simulink model "eight_model"  (R2022a)
settings: Solver=FixedStepAuto  StartTime=0.0  StopTime=10.0  FixedStep=1e-3  RelTol=1e-3  EnableMultiTasking=on
undefined symbols (not defined in the file): D0, D1, D10, D11, D12, D13, D2, D3, D4, D5, D6, D7, D8, D9, magnitude, PTA0, PTA1, PTA2, PTB23, PTB9, PTC16, PTC17, PTC2, PTC3, PTC4, PTD0, PTD1, PTD2, PTD3
libraries: etargetslib x30, frdmk64flib x18, dspstat3 x1, simulink x1
settings Model: ExtModeTrigDuration=5  Creator=12791  LastModifiedBy=12791
settings OptimizationCC: EnhancedBackFolding=on  PassReuseOutputArgsAs=Individual arguments  ZeroExternalMemoryAtStartup=off  ZeroInternalMemoryAtStartup=off  MaxStackSize=64  OptimizeBlockOrder=speed  DifferentSizesBufferReuse=on  OptimizationCustomize=off  EfficientTunableParamExpr=on
settings DebuggingCC: ParameterTunabilityLossMsg=error
settings HardwareCC: ProdBitPerPointer=32  ProdBitPerSizeT=32  ProdBitPerPtrDiffT=32  ProdLargestAtomicInteger=Long  ProdLargestAtomicFloat=Double  ProdWordSize=32  ProdHWDeviceType=ARM Compatible->ARM Cortex
settings SFSimCC: MATLABDynamicMemAlloc=off
settings RTWCC: SystemTargetFile=ert.tlc  HardwareBoard=NXP FRDM-K64F  TLCOptions="-aInlineSetEventsForThisBaseRateFcn=TLC_FALSE -aSuppressMultiTaskScheduler=TLC_FALSE  -aRateBasedStepFcn=0"  TemplateMakefile=ert_default_tmf  Toolchain=GNU Tools for ARM Embedded Processors
settings CodeAppCC: ForceParamTrailComments=on  IgnoreCustomStorageClasses=off  OperatorAnnotations=on  SimulinkDataObjDesc=on  SFDataObjDesc=on  InsertBlockDesc=on
settings ERTTargetCC: ExtModeTransport=4  ExtModeMexFile=sendToCommService

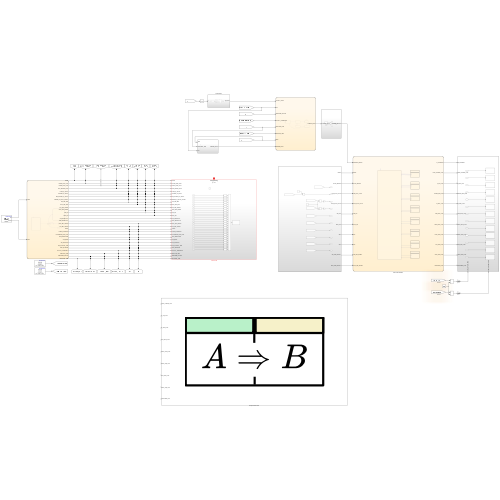
[thumbnail: Simulink's stored preview of the top-level diagram]
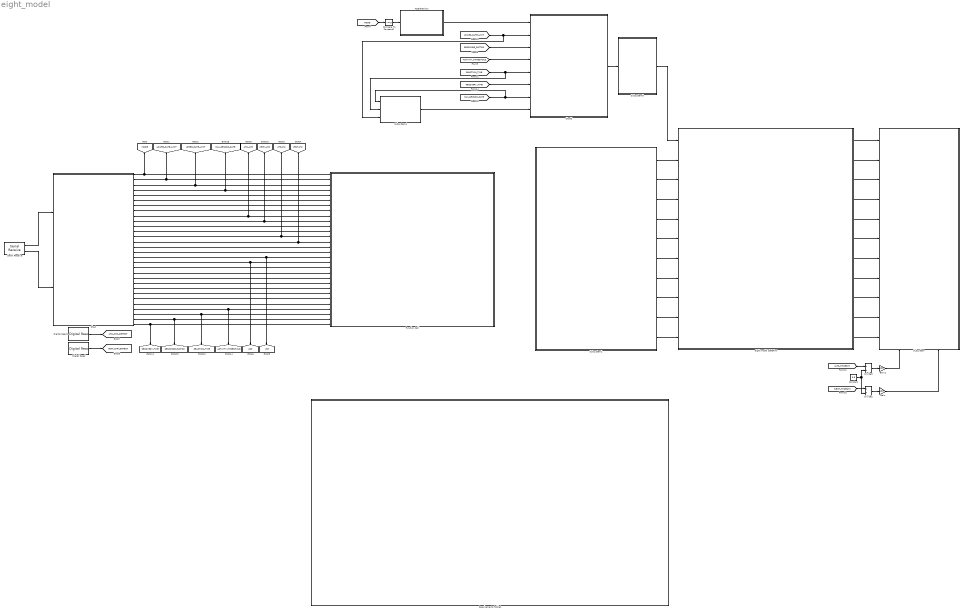
== system eight_model ==
  Acceleration1 : Subsystem
  Chart : Stateflow chart  TreatAsAtomicUnit=on
  Chart2 : Stateflow chart  TreatAsAtomicUnit=on
  Compare To Constant2 : simulink/Logic and Bit Operations/Compare To Constant  relop=>=  const=5  OutDataTypeStr=boolean
  Constant : Constant  Value=3.3
  Digital Read : frdmk64flib/Digital Read  Whichpin=PTC17 (D1)  SampleTime=-1
  Digital Read1 : frdmk64flib/Digital Read  Whichpin=PTC16 (D0)  SampleTime=-1
  Divide2 : Product  Inputs=*/
  Divide3 : Product  Inputs=*/
  Function Call : Subsystem  TreatAsAtomicUnit=on
  Gain : Gain  Gain=100
  Gain1 : Gain  Gain=100
  Requirements Table1 : Requirements Table  TreatAsAtomicUnit=on
  Serial Receive : frdmk64flib/Serial Receive  SCIModule=0  Baudrate=uint32(9600)  Parity=None  StopBits=1  HardwareFlowControl=None  ByteOrder=LittleEndian  DataType=uint8  DataLength=10  BlockingMode=off  OutputStatus=on  SampleTime=0.1
  Subsystem : Subsystem
      settings: PortSchema="{\"entries\":[{\"content\":{\"sides\":[{\"content\":{\"connectorIds\":[\"In1\",\"In2\",\"In3\",\"In4\",\"In5\",\"In6\",\"In7\",\"In8\",\"In9\",\"In10\",\"In11\"]},\"type\":\"ConnectorPlacement.EquallySpacedRectSide\",\"uuid\":\"cf431d19-a261-4061-b975-82ab8e4554ba\"},{\"content\":{\"connectorIds\":[],\"side\":\"RIGHT\"},\"type\":\"ConnectorPlacement.EquallySpacedRectSide\",\"uuid\":\"d9d96e0a-6018-4f8e-a98f-6eed3a91414e\"},{\"content\":{\"connectorIds\":[],\"side\":\"TOP\"},\"type\":\"ConnectorPlacement.EquallySpacedRectSide\",\"uuid\":\"2358aaff-c3a0-4959-bedb-835f64f1bbed\"},{\"content\":{\"connectorIds\":[\"In12\",\"In13\"],\"side\":\"BOTTOM\"},\"type\":\"ConnectorPlacement.EquallySpacedRectSide\",\"uuid\":\"ece4eb5b-308d-4002-b014-99ad51b61e06\"}]},\"type\":\"ConnectorPlacement.EquallySpacedConnector\",\"uuid\":\"cdbd5127-fb13-4f48-9ecc-e21d40fbaa52\"}],\"packageUris\":[\"http://schema.mathworks.com/mf0/Connector/R2020b\"],\"version\":\"1.0\"}"
  Subsystem1 : Subsystem
  Subsystem4 : Subsystem
  Subsystem5 : Subsystem
  eight model stateflow : Stateflow chart  TreatAsAtomicUnit=on
      settings: PortSchema="{\"entries\":[{\"content\":{\"sides\":[{\"content\":{\"connectorIds\":[\"In6\",\"In7\",\"In2\",\"In4\",\"In1\",\"In8\",\"In9\",\"In11\",\"In10\",\"In5\",\"In3\"]},\"type\":\"ConnectorPlacement.EquallySpacedRectSide\",\"uuid\":\"7bd189cb-d286-447b-b347-38d7b12e59ee\"},{\"content\":{\"connectorIds\":[\"Out1\",\"Out2\",\"Out3\",\"Out4\",\"Out5\",\"Out6\",\"Out7\",\"Out8\",\"Out9\",\"Out10\",\"Out11\"],\"side\":\"RIGHT\"},\"type\":\"ConnectorPlacement.EquallySpacedRectSide\",\"uuid\":\"522f4543-8a7d-441b-9c0c-141bccf5cf26\"},{\"content\":{\"connectorIds\":[],\"side\":\"TOP\"},\"type\":\"ConnectorPlacement.EquallySpacedRectSide\",\"uuid\":\"cf7ae06b-6ef3-498b-825a-38a0a4c90c8a\"}]},\"type\":\"ConnectorPlacement.EquallySpacedConnector\",\"uuid\":\"ae15f7ff-4998-48cc-acd9-270deb6c013f\"}],\"packageUris\":[\"http://schema.mathworks.com/mf0/Connector/R2020b\"],\"version\":\"1.0\"}"
  tag scope: ACTIVITY_THRESHOLD=global, ARP=global, ATR_AMP=global, ATR_CMP_DETECT=global, ATR_PW=global, LOWER_RATE_LIMIT=global, MAX_SENSOR_RATE=global, MODE=global, REACTION_TIME=global, RECOVERY_TIME=global, RESPONSE_FACTOR=global, UPPER_RATE_LIMIT=global, VENT_AMP=global, VENT_CMP_DETECT=global, VENT_PW=global, VRP=global
  wires:
  eight model stateflow/1(IS_CHARGING) -> Subsystem/1(IS_CHARGING)
  eight model stateflow/2(PACE_CHARGE_CTRL) -> Subsystem/2(PACE_CHARGE_CTRL)
  eight model stateflow/3(Z_ATR_CTRL) -> Subsystem/3(Z_ATR_CTRL)
  eight model stateflow/4(PACING_REF_PWM) -> Subsystem/4(PACING_REF_PWM)
  eight model stateflow/5(Z_VENT_CTRL) -> Subsystem/5(Z_VENT_CTRL)
  eight model stateflow/6(ATR_PACE_CTRL) -> Subsystem/6(ATR_PACE_CTRL)
  eight model stateflow/7(VENT_PACE_CTRL) -> Subsystem/7(VENT_PACE_CTRL)
  eight model stateflow/8(PACE_GND_CTRL) -> Subsystem/8(PACE_GND_CTRL)
  eight model stateflow/9(ATR_GND_CTRL) -> Subsystem/9(ATR_GND_CTRL)
  eight model stateflow/10(VENT_GND_CTRL) -> Subsystem/10(VENT_GND_CTRL)
  eight model stateflow/11(FRONTEND_CTRL) -> Subsystem/11(FRONTEND_CTRL)
  Serial Receive/1 -> Chart/1(rxdata)
  Serial Receive/2 -> Chart/2(status)
  Chart/1(MODE) -> Function Call/1(MODE), [MODE]
  Chart/2(LOWER_RATE_LIMIT) -> Function Call/2(LOWER_RATE_LIMIT), [LOWER_RATE_LIMIT]
  Chart/3(UPPER_RATE_LIMIT) -> Function Call/3(UPPER_RATE_LIMIT), [UPPER_RATE_LIMIT]
  Chart/4(MAX_SENSOR_RATE) -> Function Call/4(MAX_SENSOR_RATE), [MAX_SENSOR_RATE]
  Chart/5(FIXED_AV_DELAY) -> Function Call/5(FIXED_AV_DELAY)
  Chart/6(DYNAMIC_AV_DELAY) -> Function Call/6(DYNAMIC_AV_DELAY)
  Chart/7(MIN_DYNAMIC_AV_DELAY) -> Function Call/7(MIN_DYNAMIC_AV_DELAY)
  Chart/8(SENSED_AV_DELAY_OFFSET) -> Function Call/8(SENSED_AV_DELAY_OFFSET)
  Chart/11(ATR_AMP_UNREG) -> Function Call/11(ATR_AMP_UNREG)
  Chart/12(VENT_AMP_UNREG) -> Function Call/12(VENT_AMP_UNREG)
  Chart/13(ATR_PW) -> Function Call/13(ATR_PW), [ATR_PW]
  Chart/14(VENT_PW) -> Function Call/14(VENT_PW), [VENT_PW]
  Chart/15(ATR_SENSITIVITY) -> Function Call/15(ATR_SENSITIVITY)
  Chart/16(VENT_SENSITIVITY) -> Function Call/16(VENT_SENSITIVITY)
  Chart/17(VENT_REF_PERIOD) -> Function Call/17(VENT_REF_PERIOD), [VRP]
  Chart/18(ATR_REF_PERIOD) -> Function Call/18(ATR_REF_PERIOD), [ARP]
  Chart/19(PVARP) -> Function Call/19(PVARP)
  Chart/20(PVARP_EXTENSION) -> Function Call/20(PVARP_EXTENSION)
  Chart/21(HYSTERESIS_RATE_LIMIT) -> Function Call/21(HYSTERESIS_RATE_LIMIT)
  Chart/22(RATE_SMOOTHING) -> Function Call/22(RATE_SMOOTHING)
  Chart/23(ATR_MODE) -> Function Call/23(ATR_MODE)
  Chart/24(ATR_DURATION) -> Function Call/24(ATR_DURATION)
  Chart/25(ATR_FALLBACK_TIME) -> Function Call/25(ATR_FALLBACK_TIME)
  Chart/26(VENT_BLANKING) -> Function Call/26(VENT_BLANKING)
  Chart/27(ACTIVITY_THRESHOLD) -> [ACTIVITY_THRESHOLD], Function Call/27(ACTIVITY_THRESHOLD)
  Chart/29(RESPONSE_FACTOR) -> Function Call/29(RESPONSE_FACTOR), [RESPONSE_FACTOR]
  Chart/30(RECOVERY_TIME) -> Function Call/30(RECOVERY_TIME), [RECOVERY_TIME]
  Subsystem1/2(PULSE_PERIOD) -> eight model stateflow/2(PULSE_PERIOD)
  Subsystem1/1(MODE) -> eight model stateflow/7(MODE)
  Subsystem1/4(VENT_DUTY_CYCLE) -> eight model stateflow/1(VENT_DUTY_CYCLE)
  Subsystem1/5(ATR_PW) -> eight model stateflow/8(ATR_PW)
  Subsystem1/6(VENT_PW) -> eight model stateflow/9(VENT_PW)
  Subsystem1/7(ARP) -> eight model stateflow/11(ARP)
  Subsystem1/8(VRP) -> eight model stateflow/10(VRP)
  Subsystem1/3(ATR_DUTY_CYCLE) -> eight model stateflow/4(ATR_DUTY_CYCLE)
  Subsystem1/9(ATR_CMP_DETECT) -> eight model stateflow/5(ATR_CMP_DETECT)
  Subsystem1/10(VENT_CMP_DETECT) -> eight model stateflow/3(VENT_CMP_DETECT)
  Divide2/1 -> Gain/1
  Divide3/1 -> Gain1/1
  Constant/1 -> Divide2/2, Divide3/2
  [VENT_THRESH] -> Divide2/1
  [ATR_THRESH] -> Divide3/1
  Gain/1 -> Subsystem/13(VENT_CMP_REF_PWM)
  Gain1/1 -> Subsystem/12(ATR_CMP_REF_PWM)
  Digital Read1/1 -> [ATR_CMP_DETECT]
  Digital Read/1 -> [VENT_CMP_DETECT]
  Chart/10(VENT_AMP_REG) -> Function Call/10(VENT_AMP_REG), [VENT_AMP]
  Chart/9(ATR_AMP_REG) -> Function Call/9(ATR_AMP_REG), [ATR_AMP]
  Chart/28(REACTION_TIME) -> Function Call/28(REACTION_TIME), [REACTION_TIME]
  [RESPONSE_FACTOR] -> Chart2/3(RESPONSE_FACTOR)
  Chart2/1(CURRENT_RATE) -> Subsystem5/1(CURRENT_RATE)
  [LOWER_RATE_LIMIT] -> Subsystem4/3(LRL), Chart2/2(LRL)
  Subsystem4/1(DESIRED_RATE) -> Chart2/8(DESIRED_RATE)
  [REACTION_TIME] -> Subsystem4/2(RESPONSE_TIME), Chart2/5(REACTION_TIME)
  [MAX_SENSOR_RATE] -> Subsystem4/1(MSR), Chart2/7(MSR)
  [MODE] -> Compare To Constant2/1
  Compare To Constant2/1 -> Acceleration1/1(In1)
  [ACTIVITY_THRESHOLD] -> Chart2/4(ACTIVITY_THRESHOLD)
  Acceleration1/1(ACTIVITY) -> Chart2/1(ACTIVITY_LEVEL)
  [RECOVERY_TIME] -> Chart2/6(RECOVER_TIME)
  Subsystem5/1(MODIFIED_PERIOD) -> eight model stateflow/6(MODIFIED_PERIOD)

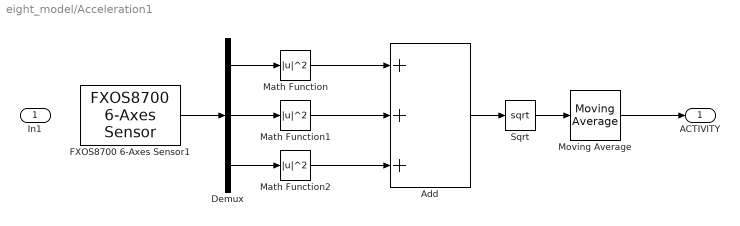
== system eight_model/Acceleration1 ==
  In1 : Inport
  Add : Sum  Inputs=+++
  Demux : Demux  Outputs=3
  FXOS8700 6-Axes Sensor1 : frdmk64flib/FXOS8700 6-Axes Sensor  Activesensor=Accelerometer only  ODR=800Hz  HybridODR=400Hz  Accelfullrange=-4g to +4g  SampleTime=-1
  Math Function : Math  Operator=magnitude^2  SignedPower=on  OutDataTypeStr=double
  Math Function1 : Math  Operator=magnitude^2  SignedPower=on  OutDataTypeStr=double
  Math Function2 : Math  Operator=magnitude^2  SignedPower=on  OutDataTypeStr=double
  Moving Average : dspstat3/Moving Average  Method=Sliding window  ForgettingFactorPort=off  SpecifyWindowLength=on  WindowLength=4  ForgettingFactor=0.9  SimulateUsing=Code generation
  Sqrt : Sqrt
  ACTIVITY : Outport  SourceOfInitialOutputValue=Input signal
  wires:
  Sqrt/1 -> Moving Average/1
  Math Function2/1 -> Add/3
  Add/1 -> Sqrt/1
  Math Function1/1 -> Add/2
  Demux/1 -> Math Function/1
  Demux/2 -> Math Function1/1
  Math Function/1 -> Add/1
  FXOS8700 6-Axes Sensor1/1 -> Demux/1
  Demux/3 -> Math Function2/1
  Moving Average/1 -> ACTIVITY/1

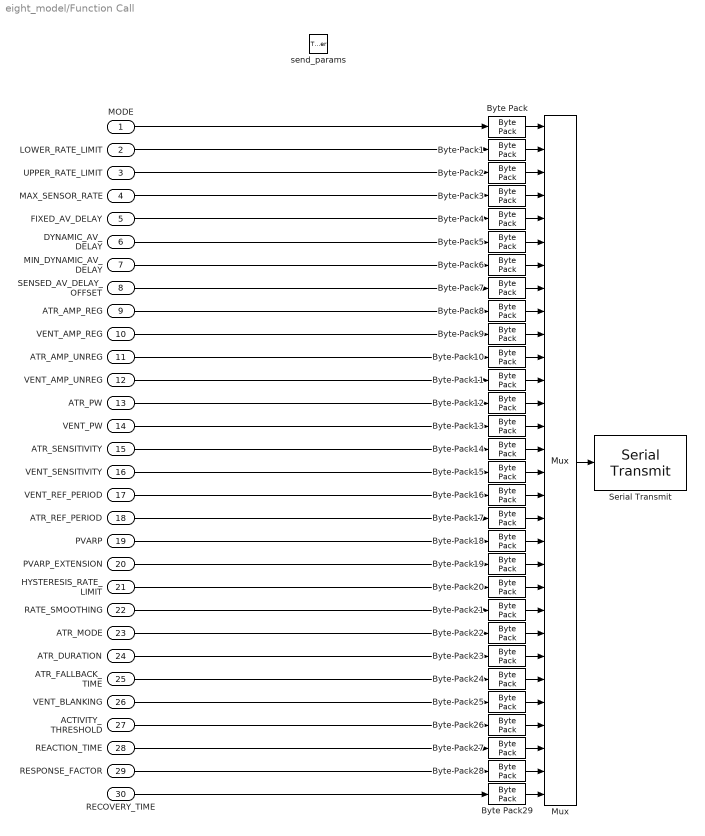
== system eight_model/Function Call ==
  MODE : Inport
  LOWER_RATE_LIMIT : Inport  Port=2
  UPPER_RATE_LIMIT : Inport  Port=3
  MAX_SENSOR_RATE : Inport  Port=4
  FIXED_AV_DELAY : Inport  Port=5
  DYNAMIC_AV_DELAY : Inport  Port=6
  MIN_DYNAMIC_AV_DELAY : Inport  Port=7
  SENSED_AV_DELAY_OFFSET : Inport  Port=8
  ATR_AMP_REG : Inport  Port=9
  VENT_AMP_REG : Inport  Port=10
  ATR_AMP_UNREG : Inport  Port=11
  VENT_AMP_UNREG : Inport  Port=12
  ATR_PW : Inport  Port=13
  VENT_PW : Inport  Port=14
  ATR_SENSITIVITY : Inport  Port=15
  VENT_SENSITIVITY : Inport  Port=16
  VENT_REF_PERIOD : Inport  Port=17
  ATR_REF_PERIOD : Inport  Port=18
  PVARP : Inport  Port=19
  PVARP_EXTENSION : Inport  Port=20
  HYSTERESIS_RATE_LIMIT : Inport  Port=21
  RATE_SMOOTHING : Inport  Port=22
  ATR_MODE : Inport  Port=23
  ATR_DURATION : Inport  Port=24
  ATR_FALLBACK_TIME : Inport  Port=25
  VENT_BLANKING : Inport  Port=26
  ACTIVITY_THRESHOLD : Inport  Port=27
  REACTION_TIME : Inport  Port=28
  RESPONSE_FACTOR : Inport  Port=29
  RECOVERY_TIME : Inport  Port=30
  send_params : TriggerPort  TriggerType=function-call  IsSimulinkFunction=on  FunctionName=send_params  VariantControl=Variant
  Byte Pack{,1..4,6..7,16..21,23..25,27..29} (19 alike) : etargetslib/Byte Pack  datatypes={'uint16'}  byteAlign=1
  Byte Pack{8..15,26} (9 alike) : etargetslib/Byte Pack  datatypes={'double'}  byteAlign=1
  Byte Pack22 : etargetslib/Byte Pack  datatypes={'boolean'}  byteAlign=1
  Byte Pack5 : etargetslib/Byte Pack  datatypes={'boolean'}  byteAlign=1
  Mux : Mux  Inputs=30
  Serial Transmit : frdmk64flib/Serial Transmit  SCIModule=0  Baudrate=uint32(9600)  Parity=None  StopBits=1  HardwareFlowControl=None  ByteOrder=LittleEndian  BlockingMode=on  OutputStatus=off
  wires:
  PVARP/1 -> Byte Pack18/1
  ATR_SENSITIVITY/1 -> Byte Pack14/1
  PVARP_EXTENSION/1 -> Byte Pack19/1
  MAX_SENSOR_RATE/1 -> Byte Pack3/1
  Byte Pack1/1 -> Mux/2
  Byte Pack7/1 -> Mux/8
  Byte Pack21/1 -> Mux/22
  ATR_AMP_UNREG/1 -> Byte Pack10/1
  Byte Pack/1 -> Mux/1
  Byte Pack20/1 -> Mux/21
  Byte Pack22/1 -> Mux/23
  Byte Pack3/1 -> Mux/4
  Byte Pack18/1 -> Mux/19
  VENT_REF_PERIOD/1 -> Byte Pack16/1
  Byte Pack17/1 -> Mux/18
  Mux/1 -> Serial Transmit/1
  Byte Pack26/1 -> Mux/27
  Byte Pack12/1 -> Mux/13
  LOWER_RATE_LIMIT/1 -> Byte Pack1/1
  RECOVERY_TIME/1 -> Byte Pack29/1
  Byte Pack9/1 -> Mux/10
  Byte Pack19/1 -> Mux/20
  Byte Pack13/1 -> Mux/14
  RESPONSE_FACTOR/1 -> Byte Pack28/1
  ATR_DURATION/1 -> Byte Pack23/1
  RATE_SMOOTHING/1 -> Byte Pack21/1
  Byte Pack8/1 -> Mux/9
  REACTION_TIME/1 -> Byte Pack27/1
  Byte Pack29/1 -> Mux/30
  Byte Pack16/1 -> Mux/17
  Byte Pack25/1 -> Mux/26
  ATR_MODE/1 -> Byte Pack22/1
  VENT_SENSITIVITY/1 -> Byte Pack15/1
  Byte Pack11/1 -> Mux/12
  VENT_PW/1 -> Byte Pack13/1
  MODE/1 -> Byte Pack/1
  VENT_AMP_REG/1 -> Byte Pack9/1
  Byte Pack24/1 -> Mux/25
  Byte Pack15/1 -> Mux/16
  Byte Pack2/1 -> Mux/3
  MIN_DYNAMIC_AV_DELAY/1 -> Byte Pack6/1
  VENT_BLANKING/1 -> Byte Pack25/1
  Byte Pack28/1 -> Mux/29
  ATR_PW/1 -> Byte Pack12/1
  FIXED_AV_DELAY/1 -> Byte Pack4/1
  VENT_AMP_UNREG/1 -> Byte Pack11/1
  Byte Pack4/1 -> Mux/5
  UPPER_RATE_LIMIT/1 -> Byte Pack2/1
  Byte Pack27/1 -> Mux/28
  SENSED_AV_DELAY_OFFSET/1 -> Byte Pack7/1
  Byte Pack6/1 -> Mux/7
  ATR_AMP_REG/1 -> Byte Pack8/1
  Byte Pack14/1 -> Mux/15
  Byte Pack10/1 -> Mux/11
  DYNAMIC_AV_DELAY/1 -> Byte Pack5/1
  Byte Pack5/1 -> Mux/6
  ATR_REF_PERIOD/1 -> Byte Pack17/1
  ACTIVITY_THRESHOLD/1 -> Byte Pack26/1
  Byte Pack23/1 -> Mux/24
  HYSTERESIS_RATE_LIMIT/1 -> Byte Pack20/1
  ATR_FALLBACK_TIME/1 -> Byte Pack24/1

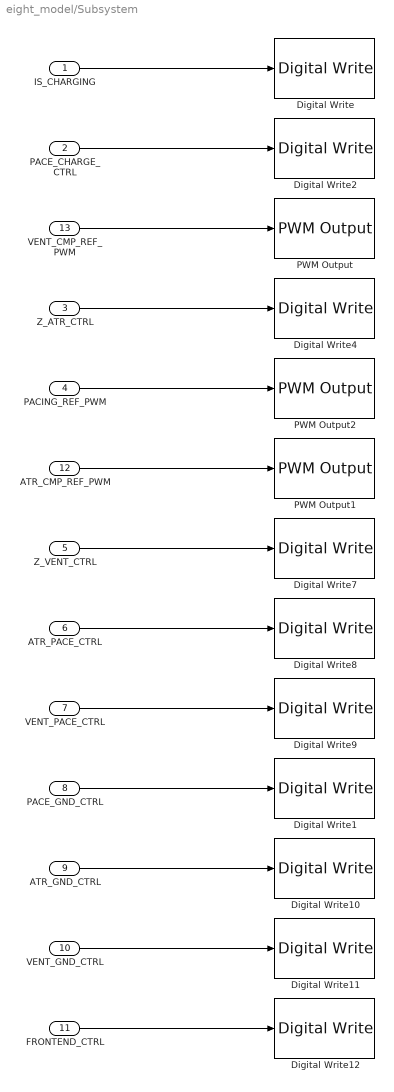
== system eight_model/Subsystem ==
  IS_CHARGING : Inport
  PACE_CHARGE_CTRL : Inport  Port=2
  Z_ATR_CTRL : Inport  Port=3
  PACING_REF_PWM : Inport  Port=4
  Z_VENT_CTRL : Inport  Port=5
  ATR_PACE_CTRL : Inport  Port=6
  VENT_PACE_CTRL : Inport  Port=7
  PACE_GND_CTRL : Inport  Port=8
  ATR_GND_CTRL : Inport  Port=9
  VENT_GND_CTRL : Inport  Port=10
  FRONTEND_CTRL : Inport  Port=11
  ATR_CMP_REF_PWM : Inport  Port=12
  VENT_CMP_REF_PWM : Inport  Port=13
  Digital Write : frdmk64flib/Digital Write  Whichpin=RED_LED
  Digital Write1 : frdmk64flib/Digital Write  Whichpin=PTD0 (D10)
  Digital Write10 : frdmk64flib/Digital Write  Whichpin=PTD2 (D11)
  Digital Write11 : frdmk64flib/Digital Write  Whichpin=PTD3 (D12)
  Digital Write12 : frdmk64flib/Digital Write  Whichpin=PTD1 (D13)
  Digital Write2 : frdmk64flib/Digital Write  Whichpin=PTB9 (D2)
  Digital Write4 : frdmk64flib/Digital Write  Whichpin=PTB23 (D4)
  Digital Write7 : frdmk64flib/Digital Write  Whichpin=PTC3 (D7)
  Digital Write8 : frdmk64flib/Digital Write  Whichpin=PTA0 (D8)
  Digital Write9 : frdmk64flib/Digital Write  Whichpin=PTC4 (D9)
  PWM Output : frdmk64flib/PWM Output  Whichpin=PTA1 (D3)  InitialFrequency=2000  InitialDutyCycle=0
  PWM Output1 : frdmk64flib/PWM Output  Whichpin=PTC2 (D6)  InitialFrequency=2000  InitialDutyCycle=0
  PWM Output2 : frdmk64flib/PWM Output  Whichpin=PTA2 (D5)  InitialFrequency=2000  InitialDutyCycle=0
  wires:
  PACE_GND_CTRL/1 -> Digital Write1/1
  Z_ATR_CTRL/1 -> Digital Write4/1
  IS_CHARGING/1 -> Digital Write/1
  PACE_CHARGE_CTRL/1 -> Digital Write2/1
  ATR_PACE_CTRL/1 -> Digital Write8/1
  Z_VENT_CTRL/1 -> Digital Write7/1
  VENT_PACE_CTRL/1 -> Digital Write9/1
  ATR_GND_CTRL/1 -> Digital Write10/1
  PACING_REF_PWM/1 -> PWM Output2/1
  VENT_CMP_REF_PWM/1 -> PWM Output/1
  ATR_CMP_REF_PWM/1 -> PWM Output1/1
  FRONTEND_CTRL/1 -> Digital Write12/1
  VENT_GND_CTRL/1 -> Digital Write11/1

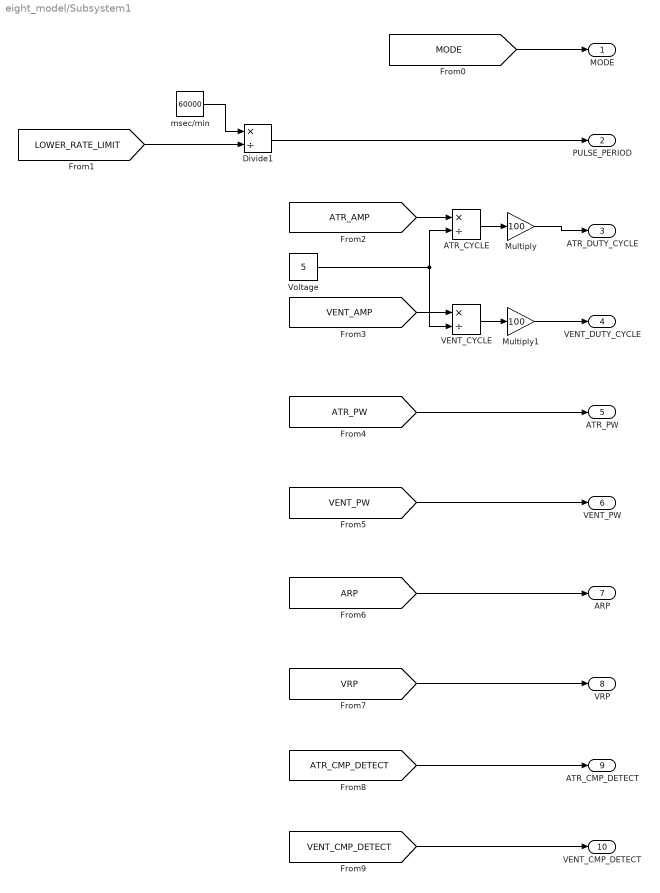
== system eight_model/Subsystem1 ==
  ATR_CYCLE : Product  Inputs=*/
  Divide1 : Product  Inputs=*/
  Multiply : Gain  Gain=100
  Multiply1 : Gain  Gain=100
  VENT_CYCLE : Product  Inputs=*/
  Voltage : Constant  Value=5
  msec/min : Constant  Value=60000  OutDataTypeStr=double  LockScale=on
  MODE : Outport
  PULSE_PERIOD : Outport  Port=2
  ATR_DUTY_CYCLE : Outport  Port=3
  VENT_DUTY_CYCLE : Outport  Port=4
  ATR_PW : Outport  Port=5
  VENT_PW : Outport  Port=6
  ARP : Outport  Port=7
  VRP : Outport  Port=8
  ATR_CMP_DETECT : Outport  Port=9
  VENT_CMP_DETECT : Outport  Port=10
  wires:
  msec/min/1 -> Divide1/1
  [LOWER_RATE_LIMIT] -> Divide1/2
  Divide1/1 -> PULSE_PERIOD/1
  Voltage/1 -> VENT_CYCLE/2, ATR_CYCLE/2
  ATR_CYCLE/1 -> Multiply/1
  VENT_CYCLE/1 -> Multiply1/1
  [MODE] -> MODE/1
  Multiply1/1 -> VENT_DUTY_CYCLE/1
  Multiply/1 -> ATR_DUTY_CYCLE/1
  [ATR_AMP] -> ATR_CYCLE/1
  [VENT_AMP] -> VENT_CYCLE/1
  [ATR_PW] -> ATR_PW/1
  [VENT_PW] -> VENT_PW/1
  [ARP] -> ARP/1
  [VRP] -> VRP/1
  [ATR_CMP_DETECT] -> ATR_CMP_DETECT/1
  [VENT_CMP_DETECT] -> VENT_CMP_DETECT/1

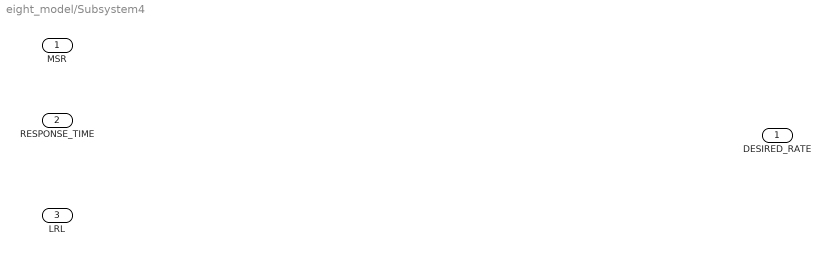
== system eight_model/Subsystem4 ==
  MSR : Inport
  RESPONSE_TIME : Inport  Port=2
  LRL : Inport  Port=3
  DESIRED_RATE : Outport

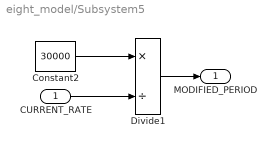
== system eight_model/Subsystem5 ==
  CURRENT_RATE : Inport
  Constant2 : Constant  Value=30000
  Divide1 : Product  Inputs=*/
  MODIFIED_PERIOD : Outport
  wires:
  CURRENT_RATE/1 -> Divide1/2
  Constant2/1 -> Divide1/1
  Divide1/1 -> MODIFIED_PERIOD/1

== stateflow chart eight_model/Chart ==
  settings: executeAtInitialization=1
  state SET_PARAM
    entry:
    MODE = 6;
    LOWER_RATE_LIMIT = typecast(rxdata(3:4), 'uint16'); % ppm
    UPPER_RATE_LIMIT = typecast(rxdata(5:6), 'uint16'); % ppm
    MAX_SENSOR_RATE = typecast(rxdata(7:8), 'uint16'); % ppm
    FIXED_AV_DELAY = typecast(rxdata(9:10), 'uint16'); % ms
    DYNAMIC_AV_DELAY = rxdata(11); % boolean
    MIN_DYNAMIC_AV_DELAY =  typecast(rxdata(12:13), 'uint16'); % ms
    SENSED_AV_DELAY_OFFSET = typecast(rxdata(14:15), 'uint16'); % ms
    ATR_AMP_REG =  typecast(rxdata(9:16), 'double'); % V
    VENT_AMP_REG = typecast(rxdata(9:16), 'double'); % V
    ATR_AMP_UNREG = typecast(rxdata(9:16), 'double'); % V
    VENT_AMP_UNREG = typecast(rxdata(9:16), 'double'); % V
    ATR_PW = typecast(rxdata(9:16), 'double'); % ms
    VENT_PW = typecast(rxdata(9:16), 'double'); % ms
    ATR_SENSITIVITY = typecast(rxdata(9:16), 'double'); % mV
    VENT_SENSITIVITY = typecast(rxdata(9:16), 'double'); % mV
    VENT_REF_PERIOD = typecast(rxdata(14:15), 'uint16'); % ms
    ATR_REF_PERIOD = typecast(rxdata(14:15), 'uint16'); % ms
    PVARP = typecast(rxdata(14:15), 'uint16'); % ms
    PVARP_EXTENSION = typecast(rxdata(14:15), 'uint16'); % ms
    HYSTERESIS_RATE_LIMIT = typecast(rxdata(14:15), 'uint16'); % ms
    RATE_SMOOTHING = typecast(rxdata(14:15), 'uint16'); % percentage
    ATR_MODE = rxdata(14); % boolean
    ATR_DURATION = typecast(rxdata(14:15), 'uint16'); % cc
    ATR_FALLBACK_TIME = typecast(rxdata(14:15), 'uint16'); % min
    VENT_BLANKING = typecast(rxdata(14:15), 'uint16'); % ms
    ACTIVITY_THRESHOLD = typecast(rxdata(14:15), 'uint16');
    REACTION_TIME = typecast(rxdata(14:15), 'uint16'); % s
    RESPONSE_FACTOR = typecast(rxdata(14:15), 'uint16');
    RECOVERY_TIME = typecast(rxdata(14:15), 'uint16'); % min
  state INITIAL
    % Set the initial values of parameters
    entry:
    MODE = 6;
    LOWER_RATE_LIMIT = 60; % ppm
    UPPER_RATE_LIMIT = 120; % ppm
    MAX_SENSOR_RATE = 120; % ppm
    FIXED_AV_DELAY = 150; % ms
    DYNAMIC_AV_DELAY = false; % boolean
    MIN_DYNAMIC_AV_DELAY = 50; % ms
    SENSED_AV_DELAY_OFFSET = 0; % ms
    ATR_AMP_REG = 3.5; % V
    VENT_AMP_REG = 3.5; % V
    ATR_AMP_UNREG = 3.75; % V
    VENT_AMP_UNREG = 3.75; % V
    ATR_PW = 0.4; % ms
    VENT_PW = 0.4; % ms
    ATR_SENSITIVITY = 0.75; % mV
    VENT_SENSITIVITY = 2.5; % mV
    VENT_REF_PERIOD = 320; % ms
    ATR_REF_PERIOD = 250; % ms
    PVARP = 250; % ms
    PVARP_EXTENSION = 0; % ms
    HYSTERESIS_RATE_LIMIT = 0; % ms
    RATE_SMOOTHING = 0; % percentage
    ATR_MODE = false; % boolean
    ATR_DURATION = 20; % cc
    ATR_FALLBACK_TIME = 1; % min
    VENT_BLANKING = 40; % ms
    ACTIVITY_THRESHOLD = 0;
    REACTION_TIME = 30; % s
    RESPONSE_FACTOR = 8;
    RECOVERY_TIME = 5; % min
  state STANDBY
    %Waiting for COM
  state ECHO_PARAM
    entry:
    send_params();
  SET_PARAM -> STANDBY
  (default) -> INITIAL
  (junction 16) -> SET_PARAM [order 1] : [rxdata(2) == hex2dec('55')]
  (junction 13) -> STANDBY [order 2]
  INITIAL -> STANDBY
  STANDBY -> (junction 13) : [status == 0]
  (junction 13) -> (junction 16) [order 1] : [rxdata(1) == hex2dec('16')]
  (junction 16) -> ECHO_PARAM [order 2] : [rxdata(2) == hex2dec('22')]
  ECHO_PARAM -> STANDBY
  data: rxdata input; status input; MODE output; LOWER_RATE_LIMIT output; UPPER_RATE_LIMIT output; MAX_SENSOR_RATE output; FIXED_AV_DELAY output; DYNAMIC_AV_DELAY output; MIN_DYNAMIC_AV_DELAY output; SENSED_AV_DELAY_OFFSET output; ATR_AMP_REG output; VENT_AMP_REG output; ATR_AMP_UNREG output; VENT_AMP_UNREG output; ATR_PW output; VENT_PW output; ATR_SENSITIVITY output; VENT_SENSITIVITY output; VENT_REF_PERIOD output; ATR_REF_PERIOD output; PVARP output; PVARP_EXTENSION output; HYSTERESIS_RATE_LIMIT output; RATE_SMOOTHING output; ATR_MODE output; ATR_DURATION output; ATR_FALLBACK_TIME output; VENT_BLANKING output; ACTIVITY_THRESHOLD output; REACTION_TIME output; RESPONSE_FACTOR output; RECOVERY_TIME output

== stateflow chart eight_model/Requirements Table1 ==
  (default) -> (junction 1073743086)
  (junction 1073743086) -> (junction 1073743087) : {
      | % SF_REQ_REV_07
      | }
  (junction 1073743087) -> (junction 1073743089) : {
      | % HEADER_ASSIGNMENTS
      |
      | }
  (junction 1073743089) -> (junction 1073743091) : {
      | % START_A_4
      | }
  (junction 1073743091) -> (junction 1073743093) : {
      | }
  (junction 1073743093) -> (junction 1073743095)
  (junction 1073743095) -> (junction 1073743097) : {
      | }
  (junction 1073743097) -> (junction 1073743099) : {
      | % END_A_4
      | }
  (junction 1073743099) -> (junction 1073743101) : {
      | % START_R_1
      | }
  (junction 1073743101) -> (junction 1073743103) : {
      | }
  (junction 1073743103) -> (junction 1073743105) : {
      |
      |
      | }
  (junction 1073743105) -> (junction 1073743107) : {
      | }
  (junction 1073743107) -> (junction 1073743109) : {
      | % START_R_7
      | }
  (junction 1073743109) -> (junction 1073743111) : {
      | }
  (junction 1073743111) -> (junction 1073743113)
  (junction 1073743113) -> (junction 1073743115) [order 1] : [(((prev(PACE_CHARGE_CTRL)) == (1))) && (((prev(Z_ATR_CTRL)) == (0))) && (((prev(Z_VENT_CTRL)) == (0))) && (((prev(ATR_PACE_CTRL)) == (0))) && (((prev(VENT_PACE_CTRL)) == (0))) && (((prev(PACE_GND_CTRL)) == (1))) && (((prev(ATR_GND_CTRL)) == (0))) && (((prev(VENT_GND_CTRL)) == (1))) && (((prev(FRONTEND_CTRL)) == (1)))]
  (junction 1073743113) -> (junction 1073743121) [order 2]
  (junction 1073743115) -> (junction 1073743117) : {
      | reqtable_postcondition((((PACE_CHARGE_CTRL) == (1))) && (((Z_ATR_CTRL) == (0))) && (((Z_VENT_CTRL) == (0))) && (((ATR_PACE_CTRL) == (0))) && (((VENT_PACE_CTRL) == (0))) && (((PACE_GND_CTRL) == (1))) && (((ATR_GND_CTRL) == (0))) && (((VENT_GND_CTRL) == (1))) && (((FRONTEND_CTRL) == (1))), 'R:1.1');
      |
      |
      | }
  (junction 1073743117) -> (junction 1073743119) : {
      | }
  (junction 1073743119) -> (junction 1073743121)
  (junction 1073743121) -> (junction 1073743123)
  (junction 1073743123) -> (junction 1073743125) : {
      | % END_R_7
      | }
  (junction 1073743125) -> (junction 1073743170) : {
      | % START_R_13
      | }
  (junction 1073743170) -> (junction 1073743172) : {
      | }
  (junction 1073743172) -> (junction 1073743174)
  (junction 1073743174) -> (junction 1073743176) [order 1] : [(((prev(PACE_CHARGE_CTRL)) == (1))) && (((prev(Z_ATR_CTRL)) == (0))) && (((prev(Z_VENT_CTRL)) == (0))) && (((prev(ATR_PACE_CTRL)) == (0))) && (((prev(VENT_PACE_CTRL)) == (0))) && (((prev(PACE_GND_CTRL)) == (1))) && (((prev(ATR_GND_CTRL)) == (0))) && (((prev(VENT_GND_CTRL)) == (1))) && (((prev(FRONTEND_CTRL)) == (1)))]
  (junction 1073743174) -> (junction 1073743182) [order 2]
  (junction 1073743176) -> (junction 1073743178) : {
      | reqtable_postcondition((((PACE_CHARGE_CTRL) == (1))) && (((Z_ATR_CTRL) == (0))) && (((Z_VENT_CTRL) == (0))) && (((ATR_PACE_CTRL) == (0))) && (((VENT_PACE_CTRL) == (0))) && (((PACE_GND_CTRL) == (1))) && (((ATR_GND_CTRL) == (0))) && (((VENT_GND_CTRL) == (1))) && (((FRONTEND_CTRL) == (1))), 'R:1.2');
      |
      |
      | }
  (junction 1073743178) -> (junction 1073743180) : {
      | }
  (junction 1073743180) -> (junction 1073743182)
  (junction 1073743182) -> (junction 1073743184)
  (junction 1073743184) -> (junction 1073743186) : {
      | % END_R_13
      | }
  (junction 1073743186) -> (junction 1073743127) : {
      | % START_R_10
      | }
  (junction 1073743127) -> (junction 1073743129) : {
      | }
  (junction 1073743129) -> (junction 1073743131)
  (junction 1073743131) -> (junction 1073743133) [order 1] : [(((prev(PACE_CHARGE_CTRL)) == (0))) && (((prev(Z_ATR_CTRL)) == (0))) && (((prev(Z_VENT_CTRL)) == (0))) && (((prev(ATR_PACE_CTRL)) == (0))) && (((prev(VENT_PACE_CTRL)) == (1))) && (((prev(PACE_GND_CTRL)) == (1))) && (((prev(ATR_GND_CTRL)) == (0))) && (((prev(VENT_GND_CTRL)) == (0))) && (((prev(FRONTEND_CTRL)) == (1)))]
  (junction 1073743131) -> (junction 1073743139) [order 2]
  (junction 1073743133) -> (junction 1073743135) : {
      | reqtable_postcondition((((PACE_CHARGE_CTRL) == (0))) && (((Z_ATR_CTRL) == (0))) && (((Z_VENT_CTRL) == (0))) && (((ATR_PACE_CTRL) == (0))) && (((VENT_PACE_CTRL) == (1))) && (((PACE_GND_CTRL) == (1))) && (((ATR_GND_CTRL) == (0))) && (((VENT_GND_CTRL) == (0))) && (((FRONTEND_CTRL) == (1))), 'R:1.3');
      |
      |
      | }
  (junction 1073743135) -> (junction 1073743137) : {
      | }
  (junction 1073743137) -> (junction 1073743139)
  (junction 1073743139) -> (junction 1073743141)
  (junction 1073743141) -> (junction 1073743161) : {
      | % END_R_10
      | }
  (junction 1073743161) -> (junction 1073743163) : {
      | % END_R_1
      | }
  data: PACE_CHARGE_CTRL input boolean; Z_ATR_CTRL input boolean; Z_VENT_CTRL input boolean; ATR_PACE_CTRL input boolean; VENT_PACE_CTRL input boolean; PACE_GND_CTRL input boolean; ATR_GND_CTRL input boolean; VENT_GND_CTRL input boolean; FRONTEND_CTRL input boolean =true

== stateflow chart eight_model/eight model stateflow ==
  state Start
  state AOO [group]
    state Charging_C22
      entry:
      PACING_REF_PWM = ATR_DUTY_CYCLE
      PACE_CHARGE_CTRL = true
      PACE_GND_CTRL = true
      ATR_PACE_CTRL = false
      Z_ATR_CTRL = false
      Z_VENT_CTRL = false
      VENT_PACE_CTRL = false
      VENT_GND_CTRL = false
      ATR_GND_CTRL = true
      % For LED testing
      IS_CHARGING = true
    state Pacing
      entry:
      PACE_CHARGE_CTRL = false
      PACE_GND_CTRL = true
      VENT_PACE_CTRL = false
      VENT_GND_CTRL = false
      Z_ATR_CTRL = false
      Z_VENT_CTRL = false
      ATR_GND_CTRL = false
      ATR_PACE_CTRL = true
      % For LED testing
      IS_CHARGING = false
    AOO.Charging_C22 -> AOO.Pacing [order 1] : [after(PULSE_PERIOD-ATR_PW,msec)]
    AOO.Pacing -> AOO.Charging_C22 : [after(ATR_PW,msec)]
  state VOO [group]
    state Charging_C22
      entry:
      PACING_REF_PWM = VENT_DUTY_CYCLE
      PACE_CHARGE_CTRL = true
      PACE_GND_CTRL = true
      VENT_PACE_CTRL = false
      Z_ATR_CTRL = false
      Z_VENT_CTRL = false
      ATR_PACE_CTRL = false
      ATR_GND_CTRL = false
      VENT_GND_CTRL = true
      % For LED testing
      IS_CHARGING = true
    state Pacing
      entry:
      PACE_CHARGE_CTRL = false
      PACE_GND_CTRL = true
      ATR_PACE_CTRL = false
      ATR_GND_CTRL = false
      Z_ATR_CTRL = false
      Z_VENT_CTRL = false
      VENT_GND_CTRL = false
      VENT_PACE_CTRL = true
      % For LED testing
      IS_CHARGING = false
    VOO.Charging_C22 -> VOO.Pacing [order 1] : [after(PULSE_PERIOD-VENT_PW,msec)]
    VOO.Pacing -> VOO.Charging_C22 : [after(VENT_PW,msec)]
  state AAI [group]
    state Charging_C22
      entry:
      PACING_REF_PWM = ATR_DUTY_CYCLE
      PACE_CHARGE_CTRL = true
      PACE_GND_CTRL = true
      ATR_PACE_CTRL = false
      Z_ATR_CTRL = false
      Z_VENT_CTRL = false
      VENT_PACE_CTRL = false
      VENT_GND_CTRL = false
      ATR_GND_CTRL = true
      % For LED testing
      IS_CHARGING = true
      FRONTEND_CTRL = true
    state Proxy
      entry:
      PACING_REF_PWM = ATR_DUTY_CYCLE
      PACE_CHARGE_CTRL = true
      PACE_GND_CTRL = true
      ATR_PACE_CTRL = false
      Z_ATR_CTRL = false
      Z_VENT_CTRL = false
      VENT_PACE_CTRL = false
      VENT_GND_CTRL = false
      ATR_GND_CTRL = true
      % For LED testing
      IS_CHARGING = true
    state Pacing
      entry:
      PACE_CHARGE_CTRL = false
      PACE_GND_CTRL = true
      VENT_PACE_CTRL = false
      VENT_GND_CTRL = false
      Z_ATR_CTRL = false
      Z_VENT_CTRL = false
      ATR_GND_CTRL = false
      ATR_PACE_CTRL = true
      % For LED testing
      IS_CHARGING = false
    AAI.Charging_C22 -> AAI.Proxy [order 1] : [ATR_CMP_DETECT ==  true]{DELAY = ARP}
    AAI.Proxy -> AAI.Charging_C22 : [after(DELAY,msec)]
    AAI.Charging_C22 -> AAI.Pacing [order 2] : [after(PULSE_PERIOD-ARP,msec)]
    AAI.Pacing -> AAI.Proxy : [after(ATR_PW,msec)]{DELAY = ARP - ATR_PW }
  state VVI [group]
    state Charging_C22
      entry:
      PACING_REF_PWM = VENT_DUTY_CYCLE
      PACE_CHARGE_CTRL = true
      PACE_GND_CTRL = true
      VENT_PACE_CTRL = false
      Z_ATR_CTRL = false
      Z_VENT_CTRL = false
      ATR_PACE_CTRL = false
      ATR_GND_CTRL = false
      VENT_GND_CTRL = true
      % For LED testing
      IS_CHARGING = true
      FRONTEND_CTRL = true
    state Proxy
      entry:
      PACING_REF_PWM = VENT_DUTY_CYCLE
      PACE_CHARGE_CTRL = true
      PACE_GND_CTRL = true
      VENT_PACE_CTRL = false
      Z_ATR_CTRL = false
      Z_VENT_CTRL = false
      ATR_PACE_CTRL = false
      ATR_GND_CTRL = false
      VENT_GND_CTRL = true
      % For LED testing
      IS_CHARGING = true
    state Pacing
      entry:
      PACE_CHARGE_CTRL = false
      PACE_GND_CTRL = true
      ATR_PACE_CTRL = false
      ATR_GND_CTRL = false
      Z_ATR_CTRL = false
      Z_VENT_CTRL = false
      VENT_GND_CTRL = false
      VENT_PACE_CTRL = true
      % For LED testing
      IS_CHARGING = false
    VVI.Charging_C22 -> VVI.Proxy [order 1] : [VENT_CMP_DETECT ==  true]{DELAY = VRP}
    VVI.Proxy -> VVI.Charging_C22 : [after(DELAY,msec)]
    VVI.Charging_C22 -> VVI.Pacing [order 2] : [after(PULSE_PERIOD-VRP,msec)]
    VVI.Pacing -> VVI.Proxy : [after(VENT_PW,msec)]{DELAY = VRP - VENT_PW }
  state AOOR [group]
    state Charging_C22
      entry:
      PACING_REF_PWM = ATR_DUTY_CYCLE
      PACE_CHARGE_CTRL = true
      PACE_GND_CTRL = true
      ATR_PACE_CTRL = false
      Z_ATR_CTRL = false
      Z_VENT_CTRL = false
      VENT_PACE_CTRL = false
      VENT_GND_CTRL = false
      ATR_GND_CTRL = true
      % For LED testing
      IS_CHARGING = true
    state Pacing
      entry:
      PACE_CHARGE_CTRL = false
      PACE_GND_CTRL = true
      VENT_PACE_CTRL = false
      VENT_GND_CTRL = false
      Z_ATR_CTRL = false
      Z_VENT_CTRL = false
      ATR_GND_CTRL = false
      ATR_PACE_CTRL = true
      % For LED testing
      IS_CHARGING = false
    AOOR.Charging_C22 -> AOOR.Pacing [order 1] : [after(MODIFIED_PERIOD-ATR_PW,msec)]
    AOOR.Pacing -> AOOR.Charging_C22 : [after(ATR_PW,msec)]
  state VOOR [group]
    state Charging_C22
      entry:
      PACING_REF_PWM = VENT_DUTY_CYCLE
      PACE_CHARGE_CTRL = true
      PACE_GND_CTRL = true
      VENT_PACE_CTRL = false
      Z_ATR_CTRL = false
      Z_VENT_CTRL = false
      ATR_PACE_CTRL = false
      ATR_GND_CTRL = false
      VENT_GND_CTRL = true
      % For LED testing
      IS_CHARGING = true
    state Pacing
      entry:
      PACE_CHARGE_CTRL = false
      PACE_GND_CTRL = true
      ATR_PACE_CTRL = false
      ATR_GND_CTRL = false
      Z_ATR_CTRL = false
      Z_VENT_CTRL = false
      VENT_GND_CTRL = false
      VENT_PACE_CTRL = true
      % For LED testing
      IS_CHARGING = false
    VOOR.Charging_C22 -> VOOR.Pacing [order 1] : [after(MODIFIED_PERIOD-VENT_PW,msec)]
    VOOR.Pacing -> VOOR.Charging_C22 : [after(VENT_PW,msec)]
  state AAIR [group]
    state Charging_C22
      entry:
      PACING_REF_PWM = ATR_DUTY_CYCLE
      PACE_CHARGE_CTRL = true
      PACE_GND_CTRL = true
      ATR_PACE_CTRL = false
      Z_ATR_CTRL = false
      Z_VENT_CTRL = false
      VENT_PACE_CTRL = false
      VENT_GND_CTRL = false
      ATR_GND_CTRL = true
      % For LED testing
      IS_CHARGING = true
      FRONTEND_CTRL = true
    state Proxy
      entry:
      PACING_REF_PWM = ATR_DUTY_CYCLE
      PACE_CHARGE_CTRL = true
      PACE_GND_CTRL = true
      ATR_PACE_CTRL = false
      Z_ATR_CTRL = false
      Z_VENT_CTRL = false
      VENT_PACE_CTRL = false
      VENT_GND_CTRL = false
      ATR_GND_CTRL = true
      % For LED testing
      IS_CHARGING = true
    state Pacing
      entry:
      PACE_CHARGE_CTRL = false
      PACE_GND_CTRL = true
      VENT_PACE_CTRL = false
      VENT_GND_CTRL = false
      Z_ATR_CTRL = false
      Z_VENT_CTRL = false
      ATR_GND_CTRL = false
      ATR_PACE_CTRL = true
      % For LED testing
      IS_CHARGING = false
    AAIR.Charging_C22 -> AAIR.Proxy [order 1] : [ATR_CMP_DETECT ==  true]{DELAY = ARP}
    AAIR.Proxy -> AAIR.Charging_C22 : [after(DELAY,msec)]
    AAIR.Charging_C22 -> AAIR.Pacing [order 2] : [after(MODIFIED_PERIOD-ARP,msec)]
    AAIR.Pacing -> AAIR.Proxy : [after(ATR_PW,msec)]{DELAY = ARP - ATR_PW }
  state VVIR [group]
    state Charging_C22
      entry:
      PACING_REF_PWM = VENT_DUTY_CYCLE
      PACE_CHARGE_CTRL = true
      PACE_GND_CTRL = true
      VENT_PACE_CTRL = false
      Z_ATR_CTRL = false
      Z_VENT_CTRL = false
      ATR_PACE_CTRL = false
      ATR_GND_CTRL = false
      VENT_GND_CTRL = true
      % For LED testing
      IS_CHARGING = true
      FRONTEND_CTRL = true
    state Proxy
      entry:
      PACING_REF_PWM = VENT_DUTY_CYCLE
      PACE_CHARGE_CTRL = true
      PACE_GND_CTRL = true
      VENT_PACE_CTRL = false
      Z_ATR_CTRL = false
      Z_VENT_CTRL = false
      ATR_PACE_CTRL = false
      ATR_GND_CTRL = false
      VENT_GND_CTRL = true
      % For LED testing
      IS_CHARGING = true
    state Pacing
      entry:
      PACE_CHARGE_CTRL = false
      PACE_GND_CTRL = true
      ATR_PACE_CTRL = false
      ATR_GND_CTRL = false
      Z_ATR_CTRL = false
      Z_VENT_CTRL = false
      VENT_GND_CTRL = false
      VENT_PACE_CTRL = true
      % For LED testing
      IS_CHARGING = false
    VVIR.Charging_C22 -> VVIR.Proxy [order 1] : [VENT_CMP_DETECT ==  true]{DELAY = VRP}
    VVIR.Proxy -> VVIR.Charging_C22 : [after(DELAY,msec)]
    VVIR.Charging_C22 -> VVIR.Pacing [order 2] : [after(MODIFIED_PERIOD-VRP,msec)]
    VVIR.Pacing -> VVIR.Proxy : [after(VENT_PW,msec)]{DELAY = VRP - VENT_PW }
  VOOR.Charging_C22 -> Start [order 2] : [MODE ~= 6]
  VVIR.Charging_C22 -> Start [order 3] : [MODE ~= 8]
  AAIR.Charging_C22 -> Start [order 3] : [MODE ~= 7]
  Start -> AOO.Charging_C22 [order 2] : [MODE == 1]
  Start -> VOO.Charging_C22 [order 1] : [MODE == 2]
  AOOR.Charging_C22 -> Start [order 2] : [MODE ~= 5]
  Start -> VVI.Charging_C22 [order 7] : [MODE == 4]
  Start -> AOOR.Charging_C22 [order 4] : [MODE == 5]
  (default) -> Start
  Start -> VOOR.Charging_C22 [order 8] : [MODE == 6]
  VVI.Charging_C22 -> Start [order 3] : [MODE ~= 4]
  Start -> AAI.Charging_C22 [order 3] : [MODE == 3]
  AAI.Charging_C22 -> Start [order 3] : [MODE ~= 3]
  AOO.Charging_C22 -> Start [order 2] : [MODE ~= 1]
  VOO.Charging_C22 -> Start [order 2] : [MODE ~= 2]
  Start -> AAIR.Charging_C22 [order 5] : [MODE == 7]
  Start -> VVIR.Charging_C22 [order 6] : [MODE == 8]
  data: IS_CHARGING output; PACE_CHARGE_CTRL output; Z_ATR_CTRL output; PACING_REF_PWM output; Z_VENT_CTRL output; ATR_PACE_CTRL output; VENT_PACE_CTRL output; PACE_GND_CTRL output; ATR_GND_CTRL output; VENT_GND_CTRL output; FRONTEND_CTRL output =true; VENT_DUTY_CYCLE input; PULSE_PERIOD input; VENT_CMP_DETECT input; DELAY local; ATR_DUTY_CYCLE input; ATR_CMP_DETECT input; MODIFIED_PERIOD input; MODE input; ATR_PW input; VENT_PW input; VRP input; ARP input

== stateflow chart eight_model/Chart2 ==
  state Start
    %Obtain desired pacing rate from activity level
    DESIRED_RATE=LRL
  state S1
    CURRENT_RATE = CURRENT_RATE + STEP_UP
  state S3
    CURRENT_RATE = DESIRED_RATE
  state S5
    CURRENT_RATE = CURRENT_RATE - STEP_DOWN
  state S4
    CURRENT_RATE = CURRENT_RATE - STEP_UP
  (default) -> Start
  S3 -> S3 [order 1] : [ACTIVITY_LEVEL>ACTIVITY_THRESHOLD]
  Start -> S1 [order 1] : [ACTIVITY_LEVEL>ACTIVITY_THRESHOLD]
  S1 -> S3 [order 2] : [CURRENT_RATE > DESIRED_RATE]
  Start -> Start [order 2] : [ACTIVITY_LEVEL<= ACTIVITY_THRESHOLD]
  S3 -> S5 [order 2] : [ACTIVITY_LEVEL<ACTIVITY_THRESHOLD]
  S1 -> S4 [order 1] : [ACTIVITY_LEVEL<ACTIVITY_THRESHOLD]
  S4 -> S1 [order 1] : [ACTIVITY_LEVEL>ACTIVITY_THRESHOLD]
  S5 -> Start : [CURRENT_RATE<=LRL]
  S4 -> S5 [order 2] : [ACTIVITY_LEVEL>=ACTIVITY_THRESHOLD]
  data: ACTIVITY_LEVEL input; LRL input; RESPONSE_FACTOR input; ACTIVITY_THRESHOLD input; REACTION_TIME input; RECOVER_TIME input; MSR input; DESIRED_RATE input; CURRENT_RATE output; STEP_DOWN local; STEP_UP local
